simulink subsystem "PvtSubSys_PLAN_ALC"  (R2020b)
settings: Solver=VariableStepAuto  StartTime=0.0  StopTime=10.0  RelTol=1e-3
undefined symbols (not defined in the file or in its folder): P_Global_WheelBase_m, P_Global_WheelTrack_m, P_PLAN_ALC_DPCConfirmTimeHMI, P_PLAN_ALC_DPCExtraMultiFrameConfirmCntDrv, P_PLAN_ALC_DPCExtraMultiFrameConfirmCntNoh, P_PLAN_ALC_DPCExtraMultiFrameConfirmCntOverTk, P_PLAN_ALC_DPCthresholdLcDrvLv1, P_PLAN_ALC_DPCthresholdLcDrvLv2, P_PLAN_ALC_DPCthresholdLcDrvLv3, P_PLAN_ALC_DynamicDPCthreshold, P_PLAN_ALC_FWheelPreTime, P_PLAN_ALC_LcCancelDPCThreshold, P_PLAN_ALC_LcCancelLaneChangeReqDspTimeCnt, P_PLAN_ALC_LcCancelRoadWidthOffset, P_PLAN_ALC_LcCancelRoadWidthOffsetForDPC, P_PLAN_ALC_LcCurvatureInhibitionValueBrkPoints, P_PLAN_ALC_LcCurvatureInhibitionValueTable, P_PLAN_ALC_LcDelayCntSetNoh, P_PLAN_ALC_LcDelayCntSetOverTk, P_PLAN_ALC_LCDeltaTmeGap, P_PLAN_ALC_LcDrv_DyDiffThreshold, P_PLAN_ALC_LcDrvHMILineValidFtime, P_PLAN_ALC_LcEnterLane_factor, P_PLAN_ALC_LcFinishDyDiffBrkPoint, P_PLAN_ALC_LcFinishDyDiffRwFactorForAP, P_PLAN_ALC_LcFinishDyDiffRwFactorForHMI, P_PLAN_ALC_LcFinishDyDiffTableValue, P_PLAN_ALC_LciDrvExistDefaultDisp, P_PLAN_ALC_LciOverTkDeltaSpdLv1, P_PLAN_ALC_LciOverTkDeltaSpdLv2, P_PLAN_ALC_LciOverTkDeltaSpdLv3, P_PLAN_ALC_LcOverTkDPCthreshold, P_PLAN_ALC_LcOverTkRearVehTTClimit, P_PLAN_ALC_NOHLcSwt, P_PLAN_ALC_NOHTurnSts, P_PLAN_ALC_OverTkCutOutDyRWFactor, P_PLAN_ALC_OveTkrSupDist, P_PLAN_ALC_PreCurvatureFactor, P_PLAN_ALC_PreCurvaturePreTime, P_PLAN_ALC_TurnLmpType, P_PLAN_ALC_vMinPreLC_Drv, P_PLAN_ALC_vMinPreLC_Noh, P_PLAN_ALC_vMinPreLC_OverTk, P_PLAN_LcCancelTestEnable, PLAN_ALC_DangerObjIndex, PLAN_ALC_LcCancelReason, PLAN_ALC_LcDecsLe, PLAN_ALC_LcDecsRi, PLAN_ALC_LcFeReason, PLAN_ALC_LcReason, PLAN_ALC_sts, PLAN_ALC_stsReason, PLAN_ALC_TurnLightReq
libraries: simulink x198, TrueDurationTime x21, RisingEdgeTimer x2, JumpDetectionUint x1
(part 1 of 4)
settings Model: Creator=GW00166368  LastModifiedBy=Cheng

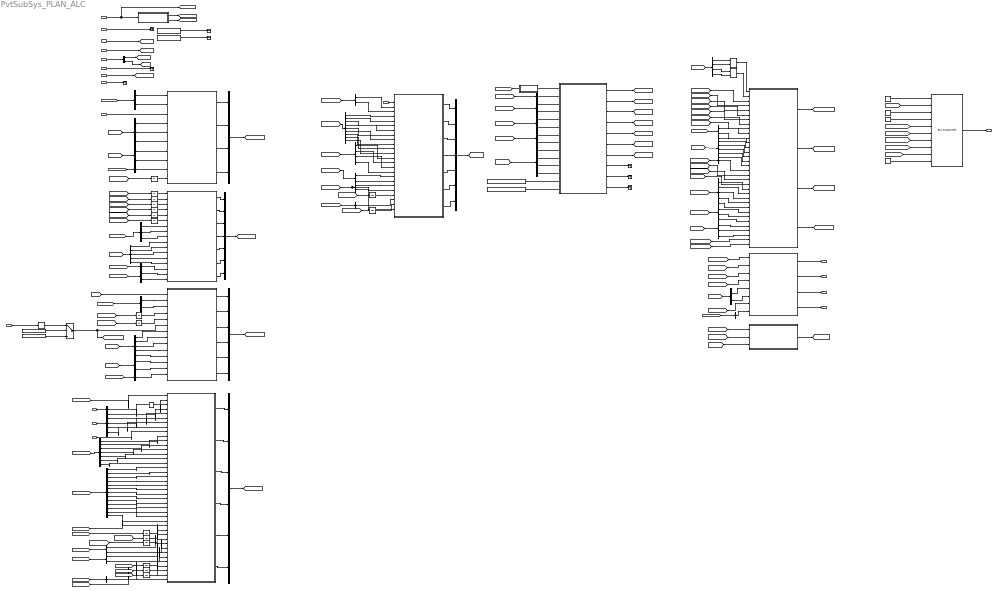
== system PvtSubSys_PLAN_ALC ==
  note: Output
      | PLAN_ALC_sts
      | 换道决策信号
      | PLAN_ALC_LcDecsLe
      | 预留
      | PLAN_ALC_LcDecsRi
      | 预留
      | PLAN_ALC_TurnLightReq
      | 转向灯请求
  UserOperation : Inport  Description=|用户操作  OutDataTypeStr=Bus: VSM_UOM_LC_BUS
  VSM_HMI : Inport  Description=|状态机状态  Port=2  OutDataTypeStr=Bus: VSM_HMI_BUS
  VSM_LON_CTRL : Inport  Description=|VSM纵向控制总线  Port=3  OutDataTypeStr=Bus: VSM_LON_CTRL_BUS
  ACC_P0 : Inport  Description=|ACCP0目标  Port=4  OutDataTypeStr=Bus: TOS_ACCP0_BUS
  PLAN_VCAN_ESP : Inport  Description=|ESP输入  Port=5  OutDataTypeStr=Bus: VCAN_ESP_MSG_BUS
  DPC_HWAinfo : Inport  Description=|DPC计算结果  Port=6  OutDataTypeStr=Bus: PLAN_DPC_ALC_BUS
  RF_input : Inport  Description=|道路融合TSR输出  Port=7
  tStartDecel : Inport  Description=s|还有多久要跟车减速  Port=8  OutDataTypeStr=single
  LSM_HWA : Inport  Description=|HWA车道线模型  Port=9  OutDataTypeStr=Bus: LSM_HWA_BUS
  LSM_PilotSts : Inport  Description=|Pilot状态 预留未使用  Port=10  OutDataTypeStr=uint8
  LSM_PilotTurnSts : Inport  Description=|换道、点灯请求  Port=11  OutDataTypeStr=uint8
  VSM_MrcReq : Inport  Description=|MRC请求  Port=12  OutDataTypeStr=uint8
  LSM_PilotRoadSts : Inport  Description=|PilotRoad状态，预留  Port=13  OutDataTypeStr=uint8
  kapTraj : Inport  Description=1/m|自车行驶预测曲率  Port=14  OutDataTypeStr=single
  ALC_DECS : Stateflow chart  TreatAsAtomicUnit=on
  AND : Logic  IconShape=distinctive  AllPortsSameDT=off  OutDataTypeStr=boolean
  AND1 : Logic  IconShape=distinctive  AllPortsSameDT=off  OutDataTypeStr=boolean
  Bus Assignment : BusAssignment  AssignedSignals=PLAN_ALC_sts,PLAN_ALC_LcDecsLe,PLAN_ALC_LcDecsRi,PLAN_ALC_TurnLightReq,PLAN_ALC_stsReason,PLAN_ALC_LcReason,PLAN_ALC_LcFeReason,PLAN_ALC_LcCancelReason,PLAN_ALC_DangerObjIndex
  Bus Selector : BusSelector  OutputSignals=ACC_SpdSetValueKmh
  Bus Selector1 : BusSelector  OutputSignals=IDP0,vxRelP0,ObjDYP0,ACCTgtObjVy,dxP0
  Bus Selector10 : BusSelector  OutputSignals=HWALineC1,HWALineC0,HWALeLineC0,HWARiLineC0,HWALeLineValid,HWARiLineValid,HWALineValid,LeLineLcAvailable,RiLineLcAvailable
  Bus Selector11 : BusSelector  OutputSignals=HWALineC0,RoadWidth,HWALeLineValid,HWARiLineValid,LeLineLcAvailable,RiLineLcAvailable
  Bus Selector12 : BusSelector  OutputSignals=LcOverTkCancelLe,LcOverTkCancelRi
  Bus Selector13 : BusSelector  OutputSignals=MLeLane,RoadWidth,HWALineValid,HWALineC3,HWALineC2,HWALineC1,HWALineC0,HWARange,preDyDiff,HWALeLineValid,HWARiLineValid,LeLineLcAvailable,RiLineLcAvailable
  Bus Selector14 : BusSelector  OutputSignals=LcCancelLe,LcCancelRi,LcFinishLe,LcFinishRi
  Bus Selector{2,15,30..32} (5 alike) : BusSelector  OutputSignals=User_LeTurnLmpOn,User_RiTurnLmpOn
  Bus Selector16 : BusSelector  OutputSignals=PLAN_ALC_LcDrvLe_LciDrv,PLAN_ALC_LcDrvRi_LciDrv,LciDrvTimeOut,LciDrvSpdLow,LciDrvSpdHigh
  Bus Selector17 : BusSelector  OutputSignals=PLAN_DPC_HWA_DangerPlaus_L,PLAN_DPC_HWA_DangerPlaus_R,PLAN_DPC_HWA_OncomingFlag_Le,PLAN_DPC_HWA_OncomingFlag_Ri
  Bus Selector18 : BusSelector  OutputSignals=preDyDiff,HWALeLineValid,HWARiLineValid
  Bus Selector{19,25,27..28} (4 alike) : BusSelector  OutputSignals=PLAN_DPC_HWA_DangerPlaus_L,PLAN_DPC_HWA_DangerPlaus_R
  Bus Selector20 : BusSelector  OutputSignals=LcDrvLe,LcDrvRi
  Bus Selector21 : BusSelector  OutputSignals=LcNohLe,LcNohRi
  Bus Selector22 : BusSelector  OutputSignals=PLAN_ALC_LcOverTkLe,PLAN_ALC_LcOverTkRi
  Bus Selector{5,9,23..24,29,39} (6 alike) : BusSelector  OutputSignals=VehSpd
  Bus Selector26 : BusSelector  OutputSignals=preDyDiff,HWALeLineValid,HWARiLineValid,LeLineLcAvailable,RiLineLcAvailable
  Bus Selector3 : BusSelector  OutputSignals=PLAN_DPC_HWA_NearestObjValid_L,PLAN_DPC_HWA_NearestObjValid_R,PLAN_DPC_HWA_NearestObjSpeed_L,PLAN_DPC_HWA_NearestObjSpeed_R,PLAN_DPC_HWA_RearObjValid,PLAN_DPC_HWA_RearObjDx,PLAN_DPC_HWA_RearObjSpeed
  Bus Selector33 : BusSelector  OutputSignals=PLAN_ALC_LcNohLe_LciNoh,PLAN_ALC_LcNohRi_LciNoh
  Bus Selector34 : BusSelector  OutputSignals=LcMrcRi
  Bus Selector35 : BusSelector  OutputSignals=LcMrcRi
  Bus Selector36 : BusSelector  OutputSignals=HWALineC0,RoadWidth
  Bus Selector37 : BusSelector  OutputSignals=HWALeLineValid,LeLineLcAvailable,HWARiLineValid,RiLineLcAvailable
  Bus Selector38 : BusSelector  OutputSignals=HWASts,NOH_Sts
  Bus Selector4 : BusSelector  OutputSignals=PLAN_DPC_HWA_DangerPlaus_L,PLAN_DPC_HWA_DangerPlaus_R,PLAN_DPC_HWA_OncomingFlag_Le,PLAN_DPC_HWA_OncomingFlag_Ri
  Bus Selector6 : BusSelector  OutputSignals=preDyDiff,HWALeLineValid,HWARiLineValid,LeLineLcAvailable,RiLineLcAvailable
  Bus Selector7 : BusSelector  OutputSignals=User_LeTurnLmpOn,User_RiTurnLmpOn,User_LC_DrvLCswt
  Bus Selector8 : BusSelector  OutputSignals=LeLineCrossing,RiLineCrossing
  Bus Creator : BusCreator  Inputs=6
  Bus Creator1 : BusCreator  Inputs=6
  Bus Creator2 : BusCreator  Inputs=7
  Bus Creator3 : BusCreator  Inputs=7
  Bus Creator4 : BusCreator  Inputs=4
  Constant : Constant  Value=P_PLAN_ALC_LcDelayCntSetNoh
  Constant1 : Constant  Value=P_PLAN_ALC_LcDelayCntSetOverTk
  Constant10 : Constant  Value=255  OutDataTypeStr=Inherit: Inherit via back propagation
  Constant2 : Constant  Value=0  OutDataTypeStr=Bus: PLAN_ALC_DECS_BUS
  Constant3 : Constant  Value=255  OutDataTypeStr=Inherit: Inherit via back propagation
  Constant4 : Constant  Value=0  OutDataTypeStr=uint8
  Constant5 : Constant  Value=11100000  OutDataTypeStr=uint32
  Constant6 : Constant  Value=0  OutDataTypeStr=Inherit: Inherit via back propagation
  Constant7 : Constant  Value=301  OutDataTypeStr=uint32
  Constant8 : Constant  Value=P_PLAN_ALC_NOHLcSwt
  Constant9 : Constant  Value=P_PLAN_ALC_NOHTurnSts  OutDataTypeStr=uint8
  Decode : Subsystem
  LC2APadapter : Subsystem
  LCCANCELadapter1 : Subsystem
  LcCancelFinishCalc1 : Subsystem
  LcDrv : Subsystem
  LcMrc : Subsystem
  LcNoh : Subsystem
  LcOverTk : Subsystem
  PLAN_IPHMI : Subsystem
  Signal Copy : SignalConversion  OverrideOpt=off
  Switch : Switch  Criteria=u2 ~= 0
  Terminator{,1..7} (8 alike) : Terminator
  Unit Delay{,1..16} (17 alike) : UnitDelay  SampleTime=-1  HasFrameUpgradeWarning=on
  WorkCond : Subsystem
  PLAN_ALC_DECS : Outport  Description=|  OutDataTypeStr=Bus: PLAN_ALC_DECS_BUS
      | PLAN决策输出：
      | PLAN_ALC_sts：1 巡航 2左换道 3右换道；
      | PLAN_ALC_LcDecsLe 不再使用；
      | PLAN_ALC_LcDecsRi 不再使用；
      | PLAN_ALC_TurnLightReq 0无请求 1左转向灯请求 2右转向灯请求 3关闭转向灯开关请求 ；
      | PLAN_ALC_stsReason HMI信号 1 换道完成请关闭转向灯 2 换道取消 3 换道超时 4 换道速度过低；
      | PLAN_ALC_LcReason 当前换道的原因；
      | PLAN_ALC_LcFeReason HMI信号 直连CAN信号HWA_LaneChangeReq用于显示箭头；
      | PLAN_ALC_LcCancelReason 换道取消的原因 bit0 驾驶员取消 bit1驾驶员取消 bit2 危险取消 bit3车道线无效取消 bit4压速换道取消
      | PLAN_ALC_DangerObjindex 不再使用；
  LC_DPC : Outport  Description=延迟换道请求DPC，用于给AP评估延迟“强度”  Port=2  OutDataTypeStr=single
  LC_Enable : Outport  Description=延迟跟车减速请求 1 有请求 0无请求  Port=3  OutDataTypeStr=boolean
  NOH_Intention : Outport  Description=NOH插空方向指示 -1左 1右 0无  Port=4  OutDataTypeStr=int8
  LaneChangeIncSetSpdReq : Outport  Description=换道加速请求 1请求 0不请求  Port=5  OutDataTypeStr=uint8
  wires:
  Signal Copy/1 -> Switch/1  "PLAN_ALC_LSMPilotTurnSts"
  Constant8/1 -> Switch/2
  LSM_PilotTurnSts/1 -> Signal Copy/1
  Constant9/1 -> Switch/3
  Constant7/1 -> Terminator7/1  "PLAN_ALC_SubModel_Number"
  Constant5/1 -> Terminator6/1  "PLAN_ALC_SubModel_VERSION"
  Bus Selector14/4 -> ALC_DECS/12(LcFinishRi)  "<LcFinishRi>"
  [LcOverTk] -> LC2APadapter/7(LcOverTk)
  PLAN_IPHMI/4(LampReq) -> [HMILampReq]
  LcDrv/6(LciDrvLe) -> Bus Creator2/6
  Constant/1 -> ALC_DECS/13(LcDelayCntSetNoh)
  [LcNoh] -> LC2APadapter/4(LcNoh)
  Decode/1(User_ALC_Swt) -> [User_ALC_Swt]
  Bus Selector30/1 -> LcCancelFinishCalc1/17(User_LeftTurnLampReq)  "<User_LeTurnLmpOn>"
  LcOverTk/6(LcOverTkRiReady) -> Bus Creator/6
  Bus Selector26/5 -> LcNoh/11(LcAvRi)  "<RiLineLcAvailable>"
  Bus Selector31/2 -> LcOverTk/35(User_RightTurnLampReq)  "<User_RiTurnLmpOn>"
  [LcNoh] -> Bus Selector33/1
  [PLAN_VCAN_ESP] -> Bus Selector29/1
  [LcReason] -> PLAN_IPHMI/5(LcReason)
  Bus Creator4/1 -> [LcMrc]
  Bus Selector28/1 -> LcOverTk/36(DPCLe)  "<PLAN_DPC_HWA_DangerPlaus_L>"
  [LcCancelInCntRi] -> Unit Delay14/1
  LcNoh/1(LcNohLe) -> Bus Creator1/1
  Bus Selector17/1 -> PLAN_IPHMI/29(DPCLe)  "<PLAN_DPC_HWA_DangerPlaus_L>"
  Constant6/1 -> Bus Assignment/10
  Bus Selector3/6 -> LcOverTk/15(Dx)  "<PLAN_DPC_HWA_RearObjDx>"
  ALC_DECS/3(LcReason) -> [LcReason]  "PLAN_ALC_LcReason"
  Bus Selector14/1 -> ALC_DECS/9(LcCancelLe)  "<LcCancelLe>"
  Unit Delay2/1 -> LcMrc/10(LcFinishInCntRi)
  Constant4/1 -> LcOverTk/2(LCKSts)
  LC2APadapter/3(NOH_Intention) -> NOH_Intention/1
  [ALC_LampReq] -> PLAN_IPHMI/34(ALC_LampReq)
  Bus Selector13/4 -> LcOverTk/20(" HWALineC3")  "<HWALineC3>"
  LSM_PilotRoadSts/1 -> Terminator5/1
  Bus Selector36/1 -> LC2APadapter/5(HWALineC0)  "<HWALineC0>"
  Bus Selector7/2 -> LcDrv/8(User_RiTurnLampON)  "<User_RiTurnLmpOn>"
  LcCancelFinishCalc1/2(LcFinishRi) -> Bus Creator3/2
  Bus Selector2/1 -> LcMrc/1(User_LeftTurnLampReq)  "<User_LeTurnLmpOn>"
  Bus Selector3/7 -> LcOverTk/16(Vx)  "<PLAN_DPC_HWA_RearObjSpeed>"
  LcMrc/4(LciMrcRi) -> Bus Creator4/4
  [LcCancelInCntLe] -> PLAN_IPHMI/8(LcCancelInCntLe)
  [ALC_sts] -> Bus Assignment/2
  Bus Selector29/1 -> LcOverTk/41(Vego_kph)  "<VehSpd>"
  [HWASts] -> WorkCond/1(HWAsts)
  Unit Delay16/1 -> LcCancelFinishCalc1/23(ALC_sts)
  Bus Assignment/1 -> PLAN_ALC_DECS/1
  VSM_LON_CTRL/1 -> Bus Selector/1
  Constant3/1 -> Bus Assignment/3  "LcDecsLe"
  [LSM_PilotTurnSts] -> LcOverTk/42(LSM_PilotTurnSts)
  [LcDrv] -> Bus Selector16/1
  LC2APadapter/4(LaneChangeIncSetSpdReq) -> LaneChangeIncSetSpdReq/1
  Bus Selector32/1 -> PLAN_IPHMI/10(UserLeTurnLamp)  "<User_LeTurnLmpOn>"
  Bus Selector13/3 -> LcOverTk/19(HWALineValid)  "<HWALineValid>"
  Bus Selector12/1 -> LcCancelFinishCalc1/2(LcOverTkCancelLe)  "<LcOverTkCancelLe>"
  Bus Selector13/5 -> LcOverTk/21(HWALineC2)  "<HWALineC2>"
  Unit Delay7/1 -> LcDrv/2(LcCancelRi)
  [LcCancelInCntLe] -> LCCANCELadapter1/1(LcCancelInCntLe)
  [NOHsts] -> LcNoh/1(NOHsts)
  Bus Selector10/8 -> LcCancelFinishCalc1/11(LeLineLcAvailable)  "<LeLineLcAvailable>"
  Bus Selector2/2 -> LcMrc/2(User_RightTurnLampReq)  "<User_RiTurnLmpOn>"
  Constant10/1 -> Bus Assignment/4  "LcDecsRi"
  [HWALine] -> Bus Selector18/1
  LcDrv/3(LciDrvSpdHigh) -> Bus Creator2/3
  LcOverTk/5(LcOverTkLeReady) -> Bus Creator/5
  ALC_DECS/1(ALC_Sts) -> [ALC_sts]  "PLAN_ALC_sts"
  Bus Creator1/1 -> [LcNoh]
  [LcOverTk] -> Bus Selector22/1
  Bus Selector3/5 -> LcOverTk/14(Valid)  "<PLAN_DPC_HWA_RearObjValid>"
  [DPC_HWAinfo] -> Bus Selector4/1
  Bus Selector1/5 -> LcOverTk/8(P0Dx)  "<dxP0>"
  Bus Selector6/4 -> LcDrv/13(LcAvLe)  "<LeLineLcAvailable>"
  Bus Selector20/1 -> ALC_DECS/3(LcfeLeDrv)  "<LcDrvLe>"
  [HWALine] -> Bus Selector36/1
  LSM_PilotSts/1 -> Terminator/1
  [LcReason] -> Unit Delay/1
  Bus Creator3/1 -> [LCCANCEL]
  Bus Selector6/5 -> LcDrv/14(LcAvRi)  "<RiLineLcAvailable>"
  Bus Selector27/1 -> LcNoh/12(DPCLe)  "<PLAN_DPC_HWA_DangerPlaus_L>"
  [LcMrc] -> Bus Selector34/1
  Bus Selector13/13 -> LcOverTk/29(LcAvRi)  "<RiLineLcAvailable>"
  [DriverLC] -> Bus Selector32/1
  Bus Selector7/1 -> LcDrv/7(User_LeTurnLampON)  "<User_LeTurnLmpOn>"
  PLAN_VCAN_ESP/1 -> [PLAN_VCAN_ESP]
  Constant1/1 -> ALC_DECS/14(LcDelayCntSetOverTk)
  [LcFinishInCntRi] -> Unit Delay11/1
  [LcCancelInCntRi] -> PLAN_IPHMI/20(LcCancelRiCnt)
  Bus Selector10/9 -> LcCancelFinishCalc1/12(RiLineLcAvailable)  "<RiLineLcAvailable>"
  Bus Selector21/2 -> ALC_DECS/6(LcfeRiPilot)  "<LcNohRi>"
  Bus Selector11/5 -> PLAN_IPHMI/16(In16)  "<LeLineLcAvailable>"
  Bus Selector16/5 -> PLAN_IPHMI/26(LciDrvSpdTooHigh)  "<LciDrvSpdHigh>"
  [LcCancelReason] -> Bus Assignment/9
  Bus Selector26/4 -> LcNoh/10(LcAvLe)  "<LeLineLcAvailable>"
  Bus Selector13/12 -> LcOverTk/28(LcAvLe)  "<LeLineLcAvailable>"
  Unit Delay3/1 -> LcDrv/3(LcFinishLe)
  [HWALine] -> LcCancelFinishCalc1/24(HWA), Bus Selector8/1
  [LcCancelInCntLe] -> Unit Delay4/1
  LcNoh/5(LcNohLeMerge) -> Bus Creator1/5
  LcDrv/2(LciDrvSpdLow) -> Bus Creator2/2
  Bus Selector36/2 -> LC2APadapter/6(RoadWidth)  "<RoadWidth>"
  Bus Selector11/6 -> PLAN_IPHMI/17(In17)  "<RiLineLcAvailable>"
  LcNoh/6(LcNohRiMerge) -> Bus Creator1/6
  Bus Selector13/10 -> LcOverTk/26(HWALineLValid)  "<HWALeLineValid>"
  LcCancelFinishCalc1/3(LcCancelLe) -> Bus Creator3/3
  Unit Delay6/1 -> LcOverTk/40(ALC_sts)
  PLAN_IPHMI/1(HMILaneChangeReq) -> [HMILaneChangeReq]
  LcOverTk/4(LcOverTkCancelRi) -> Bus Creator/4
  Unit Delay/1 -> LcOverTk/31(LcReason)
  [PLAN_VCAN_ESP] -> Bus Selector24/1
  [DriverLC] -> Bus Selector7/1
  [HWALine] -> Bus Selector13/1
  Unit Delay1/1 -> LcOverTk/32(LcCancelInCntLe)
  LcOverTk/3(LcOverTkCancelLe) -> Bus Creator/3
  WorkCond/1(Active) -> ALC_DECS/1(ActiveALC)
  Unit Delay10/1 -> LcOverTk/38(LcFinishLe)
  Bus Selector8/2 -> LcCancelFinishCalc1/20(RiLaneCross)  "<RiLineCrossing>"
  LcOverTk/1(LcOverTkLe) -> Bus Creator/1
  ALC_DECS/8(LcCntLe) -> Terminator3/1
  Bus Selector13/1 -> LcOverTk/17(DrivingOnTheMostLeftLane_b)  "<MLeLane>"
  Bus Selector32/2 -> PLAN_IPHMI/11(UserRiTurnLamp)  "<User_RiTurnLmpOn>"
  Bus Selector6/3 -> LcDrv/12(HWALineRValid)  "<HWARiLineValid>"
  Bus Selector1/4 -> LcOverTk/7(P0Vy)  "<ACCTgtObjVy>"
  [PLAN_VCAN_ESP] -> Bus Selector23/1
  Unit Delay11/1 -> LcOverTk/39(LcFinishRi)
  Unit Delay12/1 -> LcDrv/5(LcReason)
  LcMrc/1(LcMrcLe) -> Bus Creator4/1
  [DPC_HWAinfo] -> Bus Selector3/1
  Bus Selector8/1 -> LcCancelFinishCalc1/19(LeLaneCross)  "<LeLineCrossing>"
  Bus Selector13/8 -> LcOverTk/24(HWALineRange)  "<HWARange>"
  Bus Selector14/2 -> ALC_DECS/10(LcCancelRi)  "<LcCancelRi>"
  Bus Selector13/9 -> LcOverTk/25(dyDiff)  "<preDyDiff>"
  Bus Selector/1 -> LcOverTk/3(SpdSetValue_kph)  "<ACC_SpdSetValueKmh>"
  Bus Selector13/7 -> LcOverTk/23(HWALineC0)  "<HWALineC0>"
  tStartDecel/1 -> LcOverTk/9(tStartDecel)
  Bus Selector37/2 -> AND/2  "<LeLineLcAvailable>"
  Bus Selector6/1 -> LcDrv/10(dyDiff)  "<preDyDiff>"
  Bus Creator/1 -> [LcOverTk]
  Bus Selector18/1 -> LcMrc/4(dyDiff)  "<preDyDiff>"
  [DriverLC] -> Bus Selector2/1
  [ALC_sts] -> Unit Delay16/1
  [User_ALC_Swt] -> LcOverTk/30(User_ALC_Swt)
  Bus Selector13/11 -> LcOverTk/27(HWALineRValid)  "<HWARiLineValid>"
  LcDrv/7(LciDrvRi) -> Bus Creator2/7
  AND1/1 -> PLAN_IPHMI/2(RiLaneOK)
  Bus Selector1/3 -> LcOverTk/6(P0Dy)  "<ObjDYP0>"
  [LcNoh] -> Bus Selector21/1
  Bus Selector28/2 -> LcOverTk/37(DPCRi)  "<PLAN_DPC_HWA_DangerPlaus_R>"
  Bus Selector18/3 -> LcMrc/6(HWALineRValid)  "<HWARiLineValid>"
  Bus Selector13/6 -> LcOverTk/22(HWALineC1)  "<HWALineC1>"
  [LcCancelInCntRi] -> LCCANCELadapter1/2(LcCancelInCntRi)
  Bus Selector18/2 -> LcMrc/5(HWALineLValid)  "<HWALeLineValid>"
  Bus Selector3/2 -> LcOverTk/11(NearestObjValid_R)  "<PLAN_DPC_HWA_NearestObjValid_R>"
  LcDrv/5(LcDrvRi) -> Bus Creator2/5
  [HWALine] -> Bus Selector26/1
  Bus Selector10/4 -> LcCancelFinishCalc1/7(RiLineC0)  "<HWARiLineC0>"
  Bus Selector13/2 -> LcOverTk/18(LaneWidth)  "<RoadWidth>"
  VSM_MrcReq/1 -> LcMrc/3(VSM_MrcReq)  "VSM_MrcReq"
  Constant2/1 -> Bus Assignment/1
  Bus Selector19/1 -> LcMrc/7(DPCLe)  "<PLAN_DPC_HWA_DangerPlaus_L>"
  [LcReason] -> Bus Assignment/7
  LcMrc/3(LciMrcLe) -> Bus Creator4/3
  [HWALine] -> Bus Selector37/1
  LcCancelFinishCalc1/4(LcCancelRi) -> Bus Creator3/4
  Switch/1 -> LcNoh/6(LSM_PilotTurnSts), [LSM_PilotTurnSts]  "LSM_PilotTurnSts"
  DPC_HWAinfo/1 -> [DPC_HWAinfo]
  kapTraj/1 -> LcCancelFinishCalc1/1(kapTraj)
  [PLAN_VCAN_ESP] -> Bus Selector9/1
  Bus Selector9/1 -> LcMrc/9(Vego_kph)  "<VehSpd>"
  [HWALine] -> Bus Selector6/1
  Bus Selector31/1 -> LcOverTk/34(User_LeftTurnLampReq)  "<User_LeTurnLmpOn>"
  Unit Delay9/1 -> LcNoh/5(LcFinishInCntRi)
  [DPC_HWAinfo] -> Bus Selector19/1
  ALC_DECS/10(LcDelayCnt) -> Terminator2/1
  [LcFinishInCntRi] -> Unit Delay9/1
  Bus Selector10/7 -> LcCancelFinishCalc1/10(HWALineValid)  "<HWALineValid>"
  Bus Selector19/2 -> LcMrc/8(DPCRi)  "<PLAN_DPC_HWA_DangerPlaus_R>"
  ACC_P0/1 -> Bus Selector1/1
  LcMrc/2(LcMrcRi) -> Bus Creator4/2
  [LcFinishInCntLe] -> Unit Delay15/1
  Bus Selector15/1 -> LcNoh/2(User_LeftTurnLampReq)  "<User_LeTurnLmpOn>"
  Unit Delay15/1 -> LcNoh/4(LcFinishInCntLe)
  [ALC_sts] -> Unit Delay6/1
  Bus Selector10/5 -> LcCancelFinishCalc1/8(HWALineValidLe)  "<HWALeLineValid>"
  Bus Selector34/1 -> ALC_DECS/2(LcMrcRi)  "<LcMrcRi>"
  Bus Selector7/3 -> LcDrv/9(DrvLcSwt)  "<User_LC_DrvLCswt>"
  Bus Selector17/4 -> PLAN_IPHMI/32(DPC_OnComing_Ri)  "<PLAN_DPC_HWA_OncomingFlag_Ri>"
  Bus Selector37/3 -> AND1/1  "<HWARiLineValid>"
  [LCCANCEL] -> PLAN_IPHMI/21(LcCancel_Conds)
  Bus Selector33/1 -> PLAN_IPHMI/27(LciNohLe)  "<PLAN_ALC_LcNohLe_LciNoh>"
  [LcMrc] -> Bus Selector35/1
  Bus Selector37/4 -> AND1/2  "<RiLineLcAvailable>"
  [DPC_HWAinfo] -> Bus Selector17/1
  Bus Selector37/1 -> AND/1  "<HWALeLineValid>"
  Bus Selector11/3 -> PLAN_IPHMI/14(LineValidLe)  "<HWALeLineValid>"
  [DPC_HWAinfo] -> Bus Selector25/1
  Bus Selector33/2 -> PLAN_IPHMI/28(LciNohRi)  "<PLAN_ALC_LcNohRi_LciNoh>"
  [LSM_PilotTurnSts] -> PLAN_IPHMI/33(LSM_PilotTurnSts)
  Bus Selector16/2 -> PLAN_IPHMI/23(LciDrvRi)  "<PLAN_ALC_LcDrvRi_LciDrv>"
  [HWASts] -> PLAN_IPHMI/4(HWASts)
  [NOHsts] -> PLAN_IPHMI/3(NOHsts)
  Bus Selector35/1 -> PLAN_IPHMI/18(LcMrcRi)  "<LcMrcRi>"
  [HWALine] -> Bus Selector11/1
  [LcCancelInCntLe] -> PLAN_IPHMI/19(LcCancelLeCnt)
  Bus Selector16/4 -> PLAN_IPHMI/25(LciDrvSpdTooLoW)  "<LciDrvSpdLow>"
  [LcFinishInCntRi] -> PLAN_IPHMI/7(LcFinishInCntRi)
  PLAN_IPHMI/3(HMILaneChange) -> [HMILaneChange]
  [PLAN_VCAN_ESP] -> Bus Selector5/1
  Bus Selector16/3 -> PLAN_IPHMI/24(LciDrvTimeOut)  "<LciDrvTimeOut>"
  Bus Selector25/2 -> LcDrv/17(DPCRi)  "<PLAN_DPC_HWA_DangerPlaus_R>"
  Bus Creator2/1 -> [LcDrv]
  Bus Selector11/2 -> PLAN_IPHMI/13(RoadWidth)  "<RoadWidth>"
  Bus Selector4/4 -> LcCancelFinishCalc1/16(RiOnComing)  "<PLAN_DPC_HWA_OncomingFlag_Ri>"
  Bus Selector4/2 -> LcCancelFinishCalc1/14(DPCRi)  "<PLAN_DPC_HWA_DangerPlaus_R>"
  [LcReason] -> Unit Delay13/1
  Bus Selector30/2 -> LcCancelFinishCalc1/18(User_RightTurnLampReq)  "<User_RiTurnLmpOn>"
  Bus Selector10/6 -> LcCancelFinishCalc1/9(HWALineValidRi)  "<HWARiLineValid>"
  LcCancelFinishCalc1/1(LcFinishLe) -> Bus Creator3/1
  LcCancelFinishCalc1/6(LcCancelLe_Conds) -> Bus Creator3/6
  Bus Selector12/2 -> LcCancelFinishCalc1/3(LcOverTkCancelRi)  "<LcOverTkCancelRi>"
  LcCancelFinishCalc1/5(TurnLampDisable) -> Bus Creator3/5
  Bus Selector5/1 -> LcCancelFinishCalc1/22(VehSpd_Kmh)  "<VehSpd>"
  Bus Selector4/3 -> LcCancelFinishCalc1/15(LeOnComing)  "<PLAN_DPC_HWA_OncomingFlag_Le>"
  [LcFinishInCntLe] -> PLAN_IPHMI/6(LcFinishInCntLe)
  LCCANCELadapter1/1(HoldValue) -> [LcCancelReason]
  ALC_DECS/2(ALC_LampReq) -> [ALC_LampReq]
  [DriverLC] -> Bus Selector30/1
  [LcCancelInCntRi] -> PLAN_IPHMI/9(LcCancelInCntRi)
  Bus Selector10/1 -> LcCancelFinishCalc1/4(LineC1)  "<HWALineC1>"
  [HWALine] -> Bus Selector10/1
  Bus Selector1/1 -> LcOverTk/4(P0ID)  "<IDP0>"
  Bus Selector10/2 -> LcCancelFinishCalc1/5(LineC0)  "<HWALineC0>"
  LcDrv/1(LciDrvTimeOut) -> Bus Creator2/1
  LcDrv/4(LcDrvLe) -> Bus Creator2/4
  [User_DrvOverride] -> LcOverTk/1(User_DrvOverride)
  [LcFinishInCntRi] -> Unit Delay2/1
  [ALC_sts] -> Unit Delay8/1
  [HMIDispInterface] -> Bus Assignment/6
  Bus Selector11/1 -> PLAN_IPHMI/12(HWALineC0)  "<HWALineC0>"
  Bus Selector10/3 -> LcCancelFinishCalc1/6(LeLineC0)  "<HWALeLineC0>"
  UserOperation/1 -> [DriverLC], Decode/1(UserOperation)
  Bus Selector20/2 -> ALC_DECS/4(LcfeRiDrv)  "<LcDrvRi>"
  Decode/2(User_DrvOverride) -> [User_DrvOverride]
  Bus Selector16/1 -> PLAN_IPHMI/22(LciDrvLe)  "<PLAN_ALC_LcDrvLe_LciDrv>"
  AND/1 -> PLAN_IPHMI/1(LeLaneOK)
  Bus Selector17/2 -> PLAN_IPHMI/30(DPCRi)  "<PLAN_DPC_HWA_DangerPlaus_R>"
  Unit Delay14/1 -> LcOverTk/33(LcCancelInCntRi)
  [LcCancelInCntLe] -> Unit Delay1/1
  LSM_HWA/1 -> [HWALine]
  PLAN_IPHMI/2(HMIDispInterface) -> [HMIDispInterface]
  RF_input/1 -> Terminator1/1
  Bus Selector14/3 -> ALC_DECS/11(LcFinishLe)  "<LcFinishLe>"
  [HMILampReq] -> Bus Assignment/5
  Bus Selector11/4 -> PLAN_IPHMI/15(LineValidRi)  "<HWARiLineValid>"
  Unit Delay13/1 -> LcCancelFinishCalc1/21(LcReason)
  LcNoh/2(LcNohRi) -> Bus Creator1/2
  ALC_DECS/6(LcCancelCntLe) -> [LcCancelInCntLe]  "LcCancelFlagLe"
  [HMILaneChangeReq] -> Bus Assignment/8
  Bus Selector4/1 -> LcCancelFinishCalc1/13(DPCLe)  "<PLAN_DPC_HWA_DangerPlaus_L>"
  [LcDrv] -> Bus Selector20/1
  Bus Selector22/1 -> ALC_DECS/7(LcfeLeOverTk)  "<PLAN_ALC_LcOverTkLe>"
  LcNoh/4(LciNohRi) -> Bus Creator1/4
  [LCCANCEL] -> Bus Selector14/1
  [LcOverTk] -> Bus Selector12/1
  [LcCancelInCntRi] -> Unit Delay7/1
  ALC_DECS/7(LcCancelCntRi) -> [LcCancelInCntRi]  "LcCancelFlagRi"
  Bus Selector1/2 -> LcOverTk/5(P0Vr_ms)  "<vxRelP0>"
  [LcFinishInCntRi] -> Unit Delay5/1
  [LcFinishInCntLe] -> Unit Delay3/1
  Bus Selector23/1 -> LcNoh/14(Vego_kph)  "<VehSpd>"
  Bus Selector3/1 -> LcOverTk/10(NearestObjValid_L)  "<PLAN_DPC_HWA_NearestObjValid_L>"
  [ALC_sts] -> LC2APadapter/1(ALC_sts)
  Bus Selector25/1 -> LcDrv/16(DPCLe)  "<PLAN_DPC_HWA_DangerPlaus_L>"
  [LcReason] -> LC2APadapter/2(LcReason)
  Bus Selector27/2 -> LcNoh/13(DPCRi)  "<PLAN_DPC_HWA_DangerPlaus_R>"
  Bus Selector17/3 -> PLAN_IPHMI/31(DPC_OnComing_Le)  "<PLAN_DPC_HWA_OncomingFlag_Le>"
  ALC_DECS/4(LcFinishCntLe) -> [LcFinishInCntLe]  "LcFinishFlagLe"
  Bus Selector15/2 -> LcNoh/3(User_RightTurnLampReq)  "<User_RiTurnLmpOn>"
  [DriverLC] -> Bus Selector15/1
  LcNoh/3(LciNohLe) -> Bus Creator1/3
  Bus Selector6/2 -> LcDrv/11(HWALineLValid)  "<HWALeLineValid>"
  [DriverLC] -> Bus Selector31/1
  Bus Selector22/2 -> ALC_DECS/8(LcfeRiOverTk)  "<PLAN_ALC_LcOverTkRi>"
  Bus Selector3/3 -> LcOverTk/12(NearestObjSpeed_L)  "<PLAN_DPC_HWA_NearestObjSpeed_L>"
  LC2APadapter/1(LC_DPC) -> LC_DPC/1
  Unit Delay4/1 -> LcDrv/1(LcCancelLe)
  Bus Selector21/1 -> ALC_DECS/5(LcfeLePilot)  "<LcNohLe>"
  ALC_DECS/5(LcFinishCntRi) -> [LcFinishInCntRi]  "LcFinishFlagRi"
  Bus Selector24/1 -> LcDrv/15(Vego_kph)  "<VehSpd>"
  Bus Selector26/1 -> LcNoh/7(dyDiff)  "<preDyDiff>"
  LcCancelFinishCalc1/7(LcCancelRi_Conds) -> Bus Creator3/7
  [DPC_HWAinfo] -> Bus Selector27/1
  Bus Selector3/4 -> LcOverTk/13(NearestObjSpeed_R)  "<PLAN_DPC_HWA_NearestObjSpeed_R>"
  [LCCANCEL] -> LCCANCELadapter1/3(LCCANCEL)
  Bus Selector26/2 -> LcNoh/8(HWALineLValid)  "<HWALeLineValid>"
  ALC_DECS/9(LcCntRi) -> Terminator4/1
  [LcFinishInCntLe] -> Unit Delay10/1
  Unit Delay5/1 -> LcDrv/4(LcFinishRi)
  [LcReason] -> Unit Delay12/1
  VSM_HMI/1 -> Bus Selector38/1
  [DPC_HWAinfo] -> LC2APadapter/3(DPC_HWA)
  LC2APadapter/2(LC_Enable) -> LC_Enable/1
  Bus Selector26/3 -> LcNoh/9(HWALineRValid)  "<HWARiLineValid>"
  LcOverTk/2(LcOverTkRi) -> Bus Creator/2
  [DPC_HWAinfo] -> Bus Selector28/1
  Unit Delay8/1 -> LcDrv/6(ALC_sts)
  Bus Selector38/1 -> [HWASts]  "<HWASts>"
  Bus Selector38/2 -> [NOHsts]  "<NOH_Sts>"
  Bus Selector39/1 -> LC2APadapter/8(<VehSpd>)  "<VehSpd>"
  [PLAN_VCAN_ESP] -> Bus Selector39/1

== system PvtSubSys_PLAN_ALC/Decode ==
  UserOperation : Inport
  Bus Selector23 : BusSelector  OutputSignals=User_LC_ALCswt,User_LC_DrvOverride
  User_ALC_Swt : Outport
  User_DrvOverride : Outport  Port=2
  wires:
  Bus Selector23/1 -> User_ALC_Swt/1  "<User_LC_ALCswt>"
  UserOperation/1 -> Bus Selector23/1
  Bus Selector23/2 -> User_DrvOverride/1  "<User_LC_DrvOverride>"

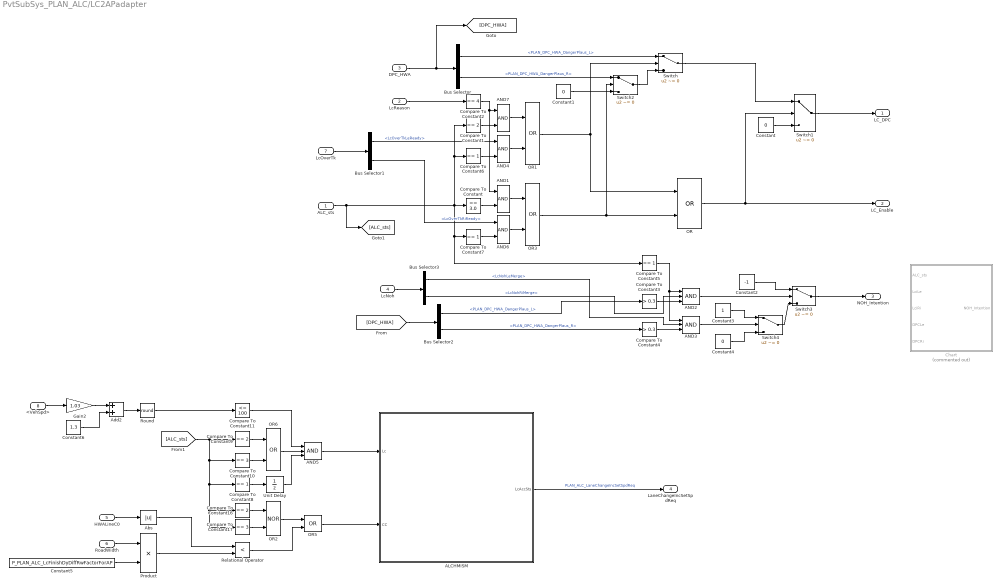
== system PvtSubSys_PLAN_ALC/LC2APadapter ==
  ALC_sts : Inport
  LcReason : Inport  Port=2
  DPC_HWA : Inport  Port=3
  LcNoh : Inport  Port=4
  HWALineC0 : Inport  Port=5
  RoadWidth : Inport  Port=6
  LcOverTk : Inport  Port=7
  <VehSpd> : Inport  Port=8
  ALCHMISM : Stateflow chart  TreatAsAtomicUnit=on
  AND{1,4,6..7} (4 alike) : Logic  AllPortsSameDT=off  OutDataTypeStr=boolean
  AND2 : Logic  Inputs=3  AllPortsSameDT=off  OutDataTypeStr=boolean
  AND3 : Logic  Inputs=3  AllPortsSameDT=off  OutDataTypeStr=boolean
  AND5 : Logic  Inputs=3  AllPortsSameDT=off  OutDataTypeStr=boolean
  Abs : Abs
  Add2 : Sum
  Bus Selector : BusSelector  OutputSignals=PLAN_DPC_HWA_DangerPlaus_L,PLAN_DPC_HWA_DangerPlaus_R
  Bus Selector1 : BusSelector  OutputSignals=LcOverTkLeReady,LcOverTkRiReady
  Bus Selector2 : BusSelector  OutputSignals=PLAN_DPC_HWA_DangerPlaus_L,PLAN_DPC_HWA_DangerPlaus_R
  Bus Selector3 : BusSelector  OutputSignals=LcNohLeMerge,LcNohRiMerge
  Chart : Stateflow chart  Commented=on  TreatAsAtomicUnit=on
  Compare To Constant : simulink/Logic and Bit Operations/Compare To Constant  relop===  const=3.0  OutDataTypeStr=boolean
  Compare To Constant1 : simulink/Logic and Bit Operations/Compare To Constant  relop===  const=2  OutDataTypeStr=boolean
  Compare To Constant10 : simulink/Logic and Bit Operations/Compare To Constant  relop===  const=3  OutDataTypeStr=boolean
  Compare To Constant11 : simulink/Logic and Bit Operations/Compare To Constant  relop=<=  const=100  OutDataTypeStr=boolean
  Compare To Constant16 : simulink/Logic and Bit Operations/Compare To Constant  relop===  const=2  OutDataTypeStr=boolean
  Compare To Constant17 : simulink/Logic and Bit Operations/Compare To Constant  relop===  const=3  OutDataTypeStr=boolean
  Compare To Constant2 : simulink/Logic and Bit Operations/Compare To Constant  relop===  const=4  OutDataTypeStr=boolean
  Compare To Constant3 : simulink/Logic and Bit Operations/Compare To Constant  relop=>  const=0.3  OutDataTypeStr=boolean
  Compare To Constant4 : simulink/Logic and Bit Operations/Compare To Constant  relop=>  const=0.3  OutDataTypeStr=boolean
  Compare To Constant{5..8} (4 alike) : simulink/Logic and Bit Operations/Compare To Constant  relop===  const=1  OutDataTypeStr=boolean
  Compare To Constant9 : simulink/Logic and Bit Operations/Compare To Constant  relop===  const=2  OutDataTypeStr=boolean
  Constant : Constant  Value=0  OutDataTypeStr=single
  Constant1 : Constant  Value=0  OutDataTypeStr=single
  Constant2 : Constant  Value=-1  OutDataTypeStr=int8
  Constant3 : Constant  OutDataTypeStr=int8
  Constant4 : Constant  Value=0  OutDataTypeStr=int8
  Constant5 : Constant  Value=P_PLAN_ALC_LcFinishDyDiffRwFactorForAP
  Constant6 : Constant  Value=1.3  OutDataTypeStr=single
  Gain2 : Gain  Gain=1.03
  OR{,1,3,5..6} (5 alike) : Logic  Operator=OR  AllPortsSameDT=off  OutDataTypeStr=boolean
  OR2 : Logic  Operator=NOR  AllPortsSameDT=off  OutDataTypeStr=boolean
  Product : Product
  Relational Operator : RelationalOperator  Operator=<  OutDataTypeStr=boolean  RndMeth=Simplest
  Round : Rounding  Operator=round
  Switch{,1..4} (5 alike) : Switch  Criteria=u2 ~= 0
  Unit Delay : UnitDelay  SampleTime=-1  HasFrameUpgradeWarning=on
  LC_DPC : Outport
  LC_Enable : Outport  Port=2
  NOH_Intention : Outport  Port=3
  LaneChangeIncSetSpdReq : Outport  Port=4
  wires:
  AND1/1 -> OR3/1
  Compare To Constant2/1 -> AND7/1, AND1/1
  AND7/1 -> OR1/1
  Bus Selector1/2 -> AND6/1  "<LcOverTkRiReady>"
  AND6/1 -> OR3/2
  Compare To Constant7/1 -> AND6/2
  Compare To Constant6/1 -> AND4/2
  AND4/1 -> OR1/2
  LcOverTk/1 -> Bus Selector1/1
  OR6/1 -> AND5/2
  Compare To Constant10/1 -> OR6/2
  Compare To Constant9/1 -> OR6/1
  AND5/1 -> ALCHMISM/1(Lc)
  ALCHMISM/1(LcAccSts) -> LaneChangeIncSetSpdReq/1  "PLAN_ALC_LaneChangeIncSetSpdReq"
  OR5/1 -> ALCHMISM/2(CC)
  Compare To Constant16/1 -> OR2/1
  Compare To Constant17/1 -> OR2/2
  Unit Delay/1 -> AND5/3
  Constant5/1 -> Product/2
  RoadWidth/1 -> Product/1
  OR2/1 -> OR5/1
  Relational Operator/1 -> OR5/2
  HWALineC0/1 -> Abs/1
  [ALC_sts] -> Compare To Constant10/1, Compare To Constant8/1, Compare To Constant16/1, Compare To Constant17/1, Compare To Constant9/1
  Compare To Constant8/1 -> Unit Delay/1
  Abs/1 -> Relational Operator/1
  Product/1 -> Relational Operator/2
  OR/1 -> Switch1/2, LC_Enable/1
  DPC_HWA/1 -> Bus Selector/1, [DPC_HWA]
  Constant/1 -> Switch1/3
  Switch/1 -> Switch1/1
  OR1/1 -> Switch/2, OR/1
  OR3/1 -> Switch2/2, OR/2
  ALC_sts/1 -> Compare To Constant/1, Compare To Constant7/1, Compare To Constant5/1, Compare To Constant6/1, Compare To Constant1/1, [ALC_sts]
  LcReason/1 -> Compare To Constant2/1
  Compare To Constant1/1 -> AND7/2
  Compare To Constant/1 -> AND1/2
  [DPC_HWA] -> Bus Selector2/1
  Switch3/1 -> NOH_Intention/1
  Switch1/1 -> LC_DPC/1
  Bus Selector/1 -> Switch/1  "<PLAN_DPC_HWA_DangerPlaus_L>"
  Bus Selector/2 -> Switch2/1  "<PLAN_DPC_HWA_DangerPlaus_R>"
  Switch2/1 -> Switch/3
  Constant1/1 -> Switch2/3
  LcNoh/1 -> Bus Selector3/1
  Bus Selector2/1 -> Compare To Constant3/1  "<PLAN_DPC_HWA_DangerPlaus_L>"
  Bus Selector2/2 -> Compare To Constant4/1  "<PLAN_DPC_HWA_DangerPlaus_R>"
  Bus Selector3/1 -> AND3/2  "<LcNohLeMerge>"
  Bus Selector3/2 -> AND2/2  "<LcNohRiMerge>"
  Compare To Constant3/1 -> AND2/3
  Compare To Constant5/1 -> AND3/1, AND2/1
  Compare To Constant4/1 -> AND3/3
  AND2/1 -> Switch3/2
  Switch4/1 -> Switch3/3
  Constant2/1 -> Switch3/1
  Constant3/1 -> Switch4/1
  AND3/1 -> Switch4/2
  Constant4/1 -> Switch4/3
  Bus Selector1/1 -> AND4/1  "<LcOverTkLeReady>"
  Compare To Constant11/1 -> AND5/1
  <VehSpd>/1 -> Gain2/1
  Round/1 -> Compare To Constant11/1
  Gain2/1 -> Add2/1
  Constant6/1 -> Add2/2
  Add2/1 -> Round/1

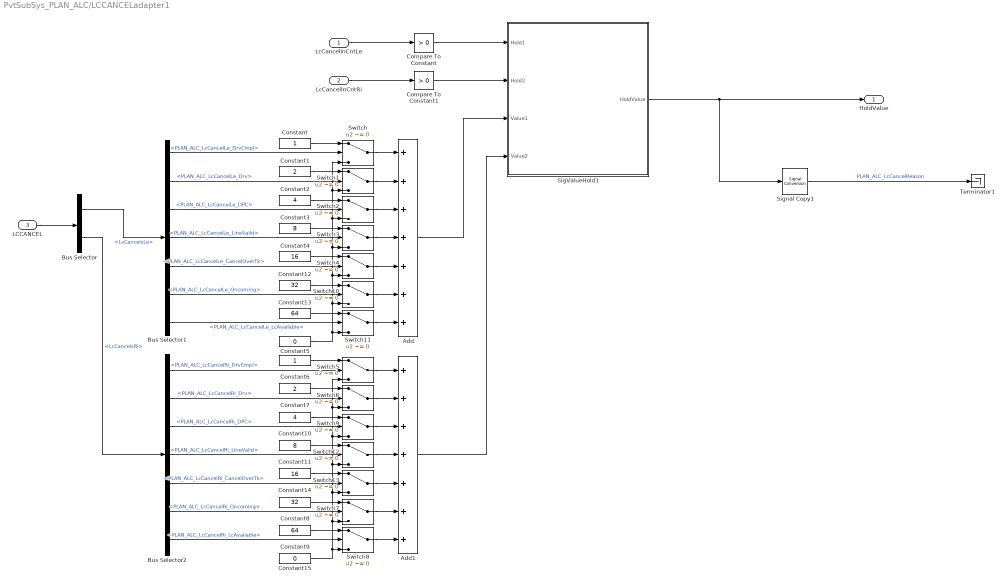
== system PvtSubSys_PLAN_ALC/LCCANCELadapter1 ==
  LcCancelInCntLe : Inport
  LcCancelInCntRi : Inport  Port=2
  LCCANCEL : Inport  Port=3
  Add : Sum  Inputs=+++++++
  Add1 : Sum  Inputs=+++++++
  Bus Selector : BusSelector  OutputSignals=LcCancelsLe,LcCancelsRi
  Bus Selector1 : BusSelector  OutputSignals=PLAN_ALC_LcCancelLe_DrvCmpl,PLAN_ALC_LcCancelLe_Drv,PLAN_ALC_LcCancelLe_DPC,PLAN_ALC_LcCancelLe_LineValid,PLAN_ALC_LcCancelLe_CancelOverTk,PLAN_ALC_LcCancelLe_Oncoming,PLAN_ALC_LcCancelLe_LcAvailable
  Bus Selector2 : BusSelector  OutputSignals=PLAN_ALC_LcCancelRi_DrvCmpl,PLAN_ALC_LcCancelRi_Drv,PLAN_ALC_LcCancelRi_DPC,PLAN_ALC_LcCancelRi_LineValid,PLAN_ALC_LcCancelRi_CancelOverTk,PLAN_ALC_LcCancelRi_Oncoming,PLAN_ALC_LcCancelRi_LcAvailable
  Compare To Constant : simulink/Logic and Bit Operations/Compare To Constant  relop=>  const=0  OutDataTypeStr=boolean
  Compare To Constant1 : simulink/Logic and Bit Operations/Compare To Constant  relop=>  const=0  OutDataTypeStr=boolean
  Constant : Constant  OutDataTypeStr=uint16
  Constant1 : Constant  Value=2  OutDataTypeStr=uint16
  Constant10 : Constant  Value=4  OutDataTypeStr=uint16
  Constant11 : Constant  Value=8  OutDataTypeStr=uint16
  Constant12 : Constant  Value=32  OutDataTypeStr=uint16
  Constant13 : Constant  Value=64  OutDataTypeStr=uint16
  Constant14 : Constant  Value=16  OutDataTypeStr=uint16
  Constant15 : Constant  Value=0  OutDataTypeStr=uint16
  Constant2 : Constant  Value=4  OutDataTypeStr=uint16
  Constant3 : Constant  Value=8  OutDataTypeStr=uint16
  Constant4 : Constant  Value=16  OutDataTypeStr=uint16
  Constant5 : Constant  Value=0  OutDataTypeStr=uint16
  Constant6 : Constant  OutDataTypeStr=uint16
  Constant7 : Constant  Value=2  OutDataTypeStr=uint16
  Constant8 : Constant  Value=32  OutDataTypeStr=uint16
  Constant9 : Constant  Value=64  OutDataTypeStr=uint16
  SigValueHold1 : Stateflow chart  TreatAsAtomicUnit=on
  Signal Copy1 : SignalConversion  OverrideOpt=off
  Switch{,1..13} (14 alike) : Switch  Criteria=u2 ~= 0
  Terminator1 : Terminator
  HoldValue : Outport
  wires:
  Add1/1 -> SigValueHold1/4(Value2)
  Add/1 -> SigValueHold1/3(Value1)
  Compare To Constant1/1 -> SigValueHold1/2(Hold2)
  Compare To Constant/1 -> SigValueHold1/1(Hold1)
  Bus Selector/2 -> Bus Selector2/1  "<LcCancelsRi>"
  Switch4/1 -> Add/5
  Switch3/1 -> Add/4
  Switch2/1 -> Add/3
  Switch1/1 -> Add/2
  Switch/1 -> Add/1
  Constant5/1 -> Switch/3, Switch1/3, Switch2/3, Switch3/3, Switch4/3, Switch10/3, Switch11/3
  Constant4/1 -> Switch4/1
  Constant3/1 -> Switch3/1
  Constant2/1 -> Switch2/1
  Constant1/1 -> Switch1/1
  Constant/1 -> Switch/1
  Bus Selector1/4 -> Switch3/2  "<PLAN_ALC_LcCancelLe_LineValid>"
  Bus Selector1/5 -> Switch4/2  "<PLAN_ALC_LcCancelLe_CancelOverTk>"
  Bus Selector1/3 -> Switch2/2  "<PLAN_ALC_LcCancelLe_DPC>"
  Bus Selector1/2 -> Switch1/2  "<PLAN_ALC_LcCancelLe_Drv>"
  Bus Selector1/1 -> Switch/2  "<PLAN_ALC_LcCancelLe_DrvCmpl>"
  Bus Selector/1 -> Bus Selector1/1  "<LcCancelsLe>"
  LcCancelInCntRi/1 -> Compare To Constant1/1
  LcCancelInCntLe/1 -> Compare To Constant/1
  LCCANCEL/1 -> Bus Selector/1
  Constant12/1 -> Switch10/1
  Bus Selector1/6 -> Switch10/2  "<PLAN_ALC_LcCancelLe_Oncoming>"
  Bus Selector1/7 -> Switch11/2  "<PLAN_ALC_LcCancelLe_LcAvailable>"
  Constant13/1 -> Switch11/1
  Switch10/1 -> Add/6
  Switch11/1 -> Add/7
  Switch8/1 -> Add1/7
  Switch7/1 -> Add1/6
  Constant9/1 -> Switch8/1
  Bus Selector2/7 -> Switch8/2  "<PLAN_ALC_LcCancelRi_LcAvailable>"
  Bus Selector2/6 -> Switch7/2  "<PLAN_ALC_LcCancelRi_Oncoming>"
  Constant8/1 -> Switch7/1
  Bus Selector2/1 -> Switch5/2  "<PLAN_ALC_LcCancelRi_DrvCmpl>"
  Bus Selector2/2 -> Switch6/2  "<PLAN_ALC_LcCancelRi_Drv>"
  Bus Selector2/3 -> Switch9/2  "<PLAN_ALC_LcCancelRi_DPC>"
  Bus Selector2/5 -> Switch13/2  "<PLAN_ALC_LcCancelRi_CancelOverTk>"
  Bus Selector2/4 -> Switch12/2  "<PLAN_ALC_LcCancelRi_LineValid>"
  Constant6/1 -> Switch5/1
  Constant7/1 -> Switch6/1
  Constant10/1 -> Switch9/1
  Constant11/1 -> Switch12/1
  Constant14/1 -> Switch13/1
  Constant15/1 -> Switch8/3, Switch7/3, Switch13/3, Switch12/3, Switch9/3, Switch6/3, Switch5/3
  Switch5/1 -> Add1/1
  Switch6/1 -> Add1/2
  Switch9/1 -> Add1/3
  Switch12/1 -> Add1/4
  Switch13/1 -> Add1/5
  SigValueHold1/1(HoldValue) -> Signal Copy1/1, HoldValue/1
  Signal Copy1/1 -> Terminator1/1  "PLAN_ALC_LcCancelReason"

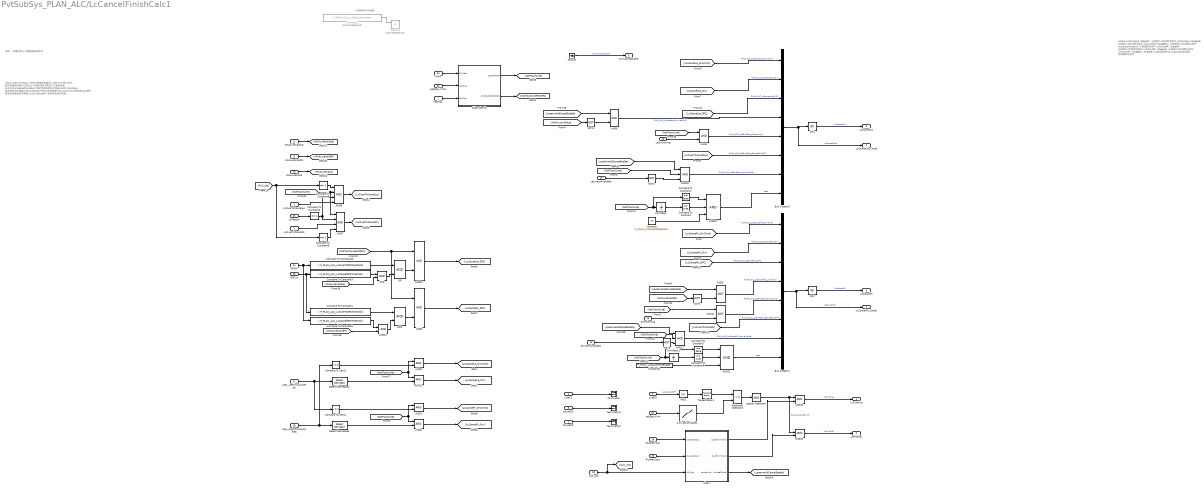
== system PvtSubSys_PLAN_ALC/LcCancelFinishCalc1 ==
  note: 关闭转向灯的系数
  note: input
      | LciDrvTimeOut 				驾驶员换道请求超时
      | LciDrvTimeOverTk			超车换道请求超时
      | DPCLe						左侧危险度
      | DPCRi						右侧危险度
      | LciDrvCompelledCancelLe		驾驶员紧急取消左换道
      | LciDrvCancelLe				驾驶员取消左换道
      | HWALineValid				HWA控制线有效性
      | LciDrvCompelledCancelRi		驾驶员紧急取消右换道
      | LciDrvCancelRi				驾驶员取消左换道
  note: output
      | LcCancelLe_StagePA		左换道P-A阶段取消条件
      | LcCancelLe_StageAB		左换道A-B阶段取消条件
      | LcCancelLe_StageBLc	左换道B-LC阶段取消条件
      | LcCancelCondsLe		左换道取消条件
      | LcCancelRi_StagePA		右换道P-A阶段取消条件
      | LcCancelRi_StageAB		右换道A-B阶段取消条件
      | LcCancelRi_StageBLc	右换道B-LC阶段取消条件
      | LcCancelCondsRi		右换道取消条件
  note: 说明：
      | 该模块用于计算换道取消条件
  kapTraj : Inport
  LcOverTkCancelLe : Inport  Port=2
  LcOverTkCancelRi : Inport  Port=3
  LineC1 : Inport  Port=4
  LineC0 : Inport  Port=5
  LeLineC0 : Inport  Port=6
  RiLineC0 : Inport  Port=7
  HWALineValidLe : Inport  Port=8
  HWALineValidRi : Inport  Port=9
  HWALineValid : Inport  Port=10
  LeLineLcAvailable : Inport  Port=11
  RiLineLcAvailable : Inport  Port=12
  DPCLe : Inport  Port=13
  DPCRi : Inport  Port=14
  LeOnComing : Inport  Port=15
  RiOnComing : Inport  Port=16
  User_LeftTurnLampReq : Inport  Port=17
  User_RightTurnLampReq : Inport  Port=18
  LeLaneCross : Inport  Port=19
  RiLaneCross : Inport  Port=20
  LcReason : Inport  Port=21
  VehSpd_Kmh : Inport  Port=22
  ALC_sts : Inport  Port=23
  HWA : Inport  Port=24
  1-D Lookup Table1 : Lookup_n-D  NumberOfTableDimensions=1  BreakpointsForDimension1=P_PLAN_ALC_LcFinishDyDiffBrkPoint  Table=P_PLAN_ALC_LcFinishDyDiffTableValue  ExtrapMethod=Clip  UseLastTableValue=on  InternalRulePriority=Speed  RndMeth=Simplest  SaturateOnIntegerOverflow=on  InputSameDT=on
  AND{,1..6,9..12,20} (12 alike) : Logic  AllPortsSameDT=off  OutDataTypeStr=boolean
  AND13 : Logic  IconShape=distinctive  AllPortsSameDT=off  OutDataTypeStr=boolean
  AND14 : Logic  IconShape=distinctive  AllPortsSameDT=off  OutDataTypeStr=boolean
  AND{15,17,19,21} (4 alike) : Logic  Inputs=3  AllPortsSameDT=off  OutDataTypeStr=boolean
  AND7 : Logic  Inputs=4  AllPortsSameDT=off  OutDataTypeStr=boolean
  AND8 : Logic  Inputs=4  AllPortsSameDT=off  OutDataTypeStr=boolean
  Abs2 : Abs
  Bus Creator3 : BusCreator  Inputs=8
  Bus Creator4 : BusCreator  Inputs=8
  Chart : Stateflow chart  TreatAsAtomicUnit=on
  Compare To Constant : simulink/Logic and Bit Operations/Compare To Constant  relop===  const=true  OutDataTypeStr=boolean
  Compare To Constant1 : simulink/Logic and Bit Operations/Compare To Constant  relop===  const=false  OutDataTypeStr=boolean
  Compare To Constant2 : simulink/Logic and Bit Operations/Compare To Constant  relop===  const=4  OutDataTypeStr=boolean
  Compare To Constant25 : simulink/Logic and Bit Operations/Compare To Constant  relop=<  const=P_PLAN_ALC_LcOverTkDPCthreshold  OutDataTypeStr=boolean
  Compare To Constant3 : simulink/Logic and Bit Operations/Compare To Constant  relop=>  const=P_PLAN_ALC_LcCancelDPCThreshold  OutDataTypeStr=boolean
  Compare To Constant4 : simulink/Logic and Bit Operations/Compare To Constant  relop=<  const=P_PLAN_ALC_LcOverTkDPCthreshold  OutDataTypeStr=boolean
  Compare To Constant5 : simulink/Logic and Bit Operations/Compare To Constant  relop=>  const=P_PLAN_ALC_LcCancelDPCThreshold  OutDataTypeStr=boolean
  Compare To Constant6 : simulink/Logic and Bit Operations/Compare To Constant  relop===  const=true  OutDataTypeStr=boolean
  Compare To Constant7 : simulink/Logic and Bit Operations/Compare To Constant  relop===  const=false  OutDataTypeStr=boolean
  Compare To Constant8 : simulink/Logic and Bit Operations/Compare To Constant  relop===  const=1  OutDataTypeStr=boolean
  Compare To Constant9 : simulink/Logic and Bit Operations/Compare To Constant  relop===  const=1  OutDataTypeStr=boolean
  Compare To Zero1 : simulink/Logic and Bit Operations/Compare To Zero  relop=~=  OutDataTypeStr=boolean
  Compare To Zero2 : simulink/Logic and Bit Operations/Compare To Zero  relop=~=  OutDataTypeStr=boolean
  Constant : Constant  Value=P_PLAN_LcCancelTestEnable
  Constant1 : Constant  Commented=on  Value=P_PLAN_ALC_LcEnterLane_factor
  Constant2 : Constant  Value=P_PLAN_LcCancelTestEnable
  Detect Decrease1 : simulink/Logic and Bit Operations/Detect Decrease  vinit=0.0  OutDataTypeStr=boolean
  Detect Decrease2 : simulink/Logic and Bit Operations/Detect Decrease  vinit=0.0  OutDataTypeStr=boolean
  Ground : Ground
  Logical Operator1 : Logic  Inputs=1  AllPortsSameDT=off  OutDataTypeStr=boolean
  NOT{1..4} (4 alike) : Logic  Operator=NOT  IconShape=distinctive  AllPortsSameDT=off  OutDataTypeStr=boolean
  OR : Logic  AllPortsSameDT=off  OutDataTypeStr=boolean
  OR1 : Logic  Operator=OR  Inputs=1  AllPortsSameDT=off  OutDataTypeStr=boolean
  OR2 : Logic  Operator=OR  Inputs=1  AllPortsSameDT=off  OutDataTypeStr=boolean
  OR3 : Logic  AllPortsSameDT=off  OutDataTypeStr=boolean
  Product1 : Product  Commented=on
  Relational Operator1 : RelationalOperator  Operator=<=  OutDataTypeStr=boolean  RndMeth=Simplest
  Subsystem3 : Subsystem
  Tapped Delay1 : simulink/Discrete/Tapped Delay  vinit=0.0  samptime=-1  NumDelays=4  DelayOrder=Oldest  includeCurrent=on
  Terminator : Terminator
  Terminator1 : Terminator
  Terminator2 : Terminator
  Unit Delay : UnitDelay  SampleTime=-1  HasFrameUpgradeWarning=on
  Unit Delay1 : UnitDelay  SampleTime=-1  HasFrameUpgradeWarning=on
  VehSpd_Kmh1 : InportShadow  Port=22
  LcFinishLe : Outport
  LcFinishRi : Outport  Port=2
  LcCancelLe : Outport  Port=3
  LcCancelRi : Outport  Port=4
  TurnLampDisable : Outport  Port=5
  LcCancelLe_Conds : Outport  Port=6
  LcCancelRi_Conds : Outport  Port=7
  wires:
  [HWALineValidLe] -> NOT4/1
  NOT4/1 -> AND6/2
  [LaneInvalidCancelEnable] -> AND6/1
  Compare To Constant8/1 -> AND8/1
  Compare To Constant9/1 -> AND7/4
  [ALC_sts] -> Compare To Constant8/1, Compare To Constant9/1
  AND21/1 -> Bus Creator4/8  "test"
  [NotTouchLine] -> Compare To Constant7/1, Unit Delay1/1
  Unit Delay1/1 -> Compare To Constant6/1
  Compare To Constant7/1 -> AND21/1
  Compare To Constant6/1 -> AND21/2
  Constant2/1 -> AND21/3
  Constant/1 -> AND19/3
  AND19/1 -> Bus Creator3/8  "test"
  Compare To Constant/1 -> AND19/2
  Compare To Constant1/1 -> AND19/1
  Unit Delay/1 -> Compare To Constant/1
  [NotTouchLine] -> Unit Delay/1, Compare To Constant1/1
  HWA/1 -> Subsystem3/1(PP_Path)
  [LaneInvalidCancelEnable] -> AND5/1
  NOT1/1 -> AND5/2
  AND14/1 -> LcFinishRi/1  "LcFinishRi"
  AND13/1 -> LcFinishLe/1  "LcFinishLe"
  Abs2/1 -> Tapped Delay1/1
  Relational Operator1/1 -> Logical Operator1/1
  1-D Lookup Table1/1 -> Relational Operator1/2
  VehSpd_Kmh/1 -> 1-D Lookup Table1/1
  Ground/1 -> TurnLampDisable/1  "TurnLampDisable"
  [NotTouchLine] -> AND4/1
  [NotTouchLine] -> AND11/1
  LineC0/1 -> Abs2/1  "LcLineDisDiff"
  LeLineC0/1 -> Terminator1/1
  RiLineC0/1 -> Terminator2/1
  Tapped Delay1/1 -> Relational Operator1/1
  LineC1/1 -> Terminator/1
  [HWALineValidRi] -> NOT1/1
  Compare To Constant5/1 -> AND12/1
  [HWALineValidRi] -> AND12/2
  AND12/1 -> OR3/2
  AND/1 -> OR/2
  [HWALineValidLe] -> AND/2
  HWALineValid/1 -> [HWALineValid]
  DPCRi/1 -> Compare To Constant5/1, Compare To Constant25/1
  [NotTouchLine] -> AND2/1, AND1/1
  OR2/1 -> LcCancelRi/1  "LcCancelRi"
  OR1/1 -> LcCancelLe/1  "LcCancelLe"
  Subsystem3/1(OutTarPath) -> [NotTouchLine]
  Logical Operator1/1 -> AND13/1, AND14/1  "PLAN_ALC_LcFinish"
  Bus Creator3/1 -> LcCancelLe_Conds/1, OR1/1  "LcCancelsLe"
  Bus Creator4/1 -> LcCancelRi_Conds/1, OR2/1  "LcCancelsRi"
  [LcCancelRi_DrvCmpl] -> Bus Creator4/1  "PLAN_ALC_LcCancelRi_DrvCmpl"
  [LcCancelLe_DrvCmpl] -> Bus Creator3/1  "PLAN_ALC_LcCancelLe_DrvCmpl"
  [LcCancelLe_Drv] -> Bus Creator3/2  "PLAN_ALC_LcCancelLe_Drv"
  [LcCancelRi_DPC] -> Bus Creator4/3  "PLAN_ALC_LcCancelRi_DPC"
  [LcCancelRi_Drv] -> Bus Creator4/2  "PLAN_ALC_LcCancelRi_Drv"
  AND6/1 -> Bus Creator3/4  "PLAN_ALC_LcCancelLe_LineValid"
  [LcCancelLe_DPC] -> Bus Creator3/3  "PLAN_ALC_LcCancelLe_DPC"
  AND5/1 -> Bus Creator4/4  "PLAN_ALC_LcCancelRi_LineValid"
  Constant1/1 -> Product1/1
  HWALineValidLe/1 -> [HWALineValidLe]
  HWALineValidRi/1 -> [HWALineValidRi]
  Compare To Zero1/1 -> AND1/2
  Detect Decrease1/1 -> AND2/2
  User_LeftTurnLampReq/1 -> Compare To Zero1/1, Detect Decrease2/1
  LeOnComing/1 -> AND4/2
  Compare To Constant25/1 -> OR/1
  OR/1 -> AND20/2
  LcReason/1 -> Compare To Constant2/1
  LcOverTkCancelRi/1 -> AND7/3
  LcOverTkCancelLe/1 -> AND8/4
  Compare To Constant2/1 -> AND7/2, AND8/3
  [NotTouchLine] -> AND8/2, AND7/1
  AND8/1 -> [LcOverTkCancelLe]
  AND7/1 -> [LcOverTkCancelRi]
  [LcOverTkCancelLe] -> Bus Creator3/6  "PLAN_ALC_LcCancelLe_CancelOverTk"
  [LcOverTkCancelRi] -> Bus Creator4/6  "PLAN_ALC_LcCancelRi_CancelOverTk"
  Compare To Constant3/1 -> AND/1
  DPCLe/1 -> Compare To Constant4/1, Compare To Constant3/1
  AND20/1 -> [LcCancelLe_DPC]
  AND3/1 -> [LcCancelRi_DPC]
  [NotTouchLineForDPC] -> AND20/1, AND3/1
  OR3/1 -> AND3/2
  Compare To Constant4/1 -> OR3/1
  Detect Decrease2/1 -> AND10/2
  Compare To Zero2/1 -> AND9/2
  [NotTouchLine] -> AND10/1, AND9/1
  User_RightTurnLampReq/1 -> Compare To Zero2/1, Detect Decrease1/1
  AND9/1 -> [LcCancelLe_DrvCmpl]
  AND10/1 -> [LcCancelLe_Drv]
  AND1/1 -> [LcCancelRi_DrvCmpl]
  AND2/1 -> [LcCancelRi_Drv]
  AND4/1 -> Bus Creator3/5  "PLAN_ALC_LcCancelLe_Oncoming"
  RiOnComing/1 -> AND11/2
  AND11/1 -> Bus Creator4/5  "PLAN_ALC_LcCancelRi_Oncoming"
  LeLaneCross/1 -> Chart/1(LeLaneCross)
  ALC_sts/1 -> Chart/3(ALC_sts), [ALC_sts]
  RiLaneCross/1 -> Chart/2(RiLaneCross)
  Chart/1(LeLcFinishValid) -> AND13/2
  Chart/2(RiLcFinishValid) -> AND14/2
  Chart/3(LaneInvalidCancelEnable) -> [LaneInvalidCancelEnable]
  kapTraj/1 -> Subsystem3/3(kapTraj)
  VehSpd_Kmh1/1 -> Subsystem3/2(VehSpd)
  LeLineLcAvailable/1 -> NOT2/1
  [NotTouchLine] -> AND15/2
  NOT2/1 -> AND15/3
  AND15/1 -> Bus Creator3/7  "PLAN_ALC_LcCancelLe_LcAvailable"
  NOT3/1 -> AND17/3
  [NotTouchLine] -> AND17/2
  RiLineLcAvailable/1 -> NOT3/1
  AND17/1 -> Bus Creator4/7  "PLAN_ALC_LcCancelRi_LcAvailable"
  Subsystem3/2(OutTarPathforDPC) -> [NotTouchLineForDPC]
  [LaneInvalidCancelEnable] -> AND15/1
  [LaneInvalidCancelEnable] -> AND17/1
